simulink model "mytest"  (R2020b)
settings: Solver=VariableStepAuto  StartTime=0.0  StopTime=10.0  RelTol=1e-3
settings Model: Creator=huang  LastModifiedBy=huang

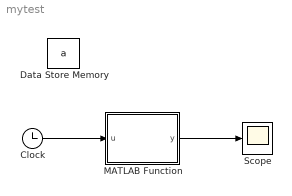
== system mytest ==
  Clock : Clock
  Data Store Memory : DataStoreMemory  DataStoreName=a  ReadBeforeWriteMsg=warning  WriteAfterWriteMsg=warning  WriteAfterReadMsg=warning  InitialValue=[1,1,1]  ShowAdditionalParam=off  OutDataTypeStr=double
  MATLAB Function : MATLAB Function  TreatAsAtomicUnit=on
  Scope : Scope
  wires:
  MATLAB Function/1(y) -> Scope/1
  Clock/1 -> MATLAB Function/1(u)

== matlab function mytest/MATLAB Function ==
  data: u input; y output; a data_store_memory
function y = fcn(u)
    global a
    a(2)=a(2)+1;
    y=a(2);
end
